simulink model "Heart_43N54P11VM_allData"  (R2023b)
settings: Solver=ode1  StartTime=0.0  StopTime=30.0  FixedStep=0.5e-3  RelTol=1e-3
model workspace: external: MAT-File C:\Users\wai484\OneDrive - The University of Auckland\Documents\HeartModelPub\models_refine\N3Data_second_43N54P11VM.mat (data not in the file)
libraries: Libs_second x152
(part 3 of 3)

== stateflow chart Heart_43N54P11VM_allData/cfgs ==
  settings: executeAtInitialization=1
  state Ini
  (default) -> Ini : {Heart=cfgdata_second; Sensing=Scfgf;}
  data: Scfg function_output; Heart output; cfgdata_second parameter; Sensing output
  function Scfg= Scfgf:
    | function Scfg= Scfgf
    | 
    | %% desired
    | xa=1;
    | xc=0.05;
    | xc1=0.1;
    | xd=1;
    | xe=0.1;
    | avd=100;
    | vad=100;
    | uni_a=1;
    | Sens_a=0.6;
    | Amp_ap=500;
    | uni_v=1;
    | Sens_v=2.8;
    | Amp_vp=500;
    | 
    | Scfg=[xa xc xc1 xd xe avd vad uni_a Sens_a Amp_ap uni_v Sens_v Amp_vp]';
    | 
    | end
